simulink model "MODELO_FUZZY"  (R2025b)
settings: Solver=VariableStepAuto  StartTime=0.0  StopTime=30000  RelTol=1e-3
libraries: fuzblock x1
settings Model: PacingRate=1000  Creator=Usuario  LastModifiedBy=Usuario

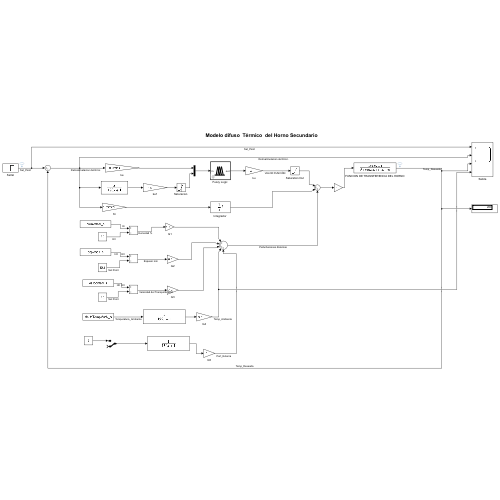
[thumbnail: Simulink's stored preview of the top-level diagram]
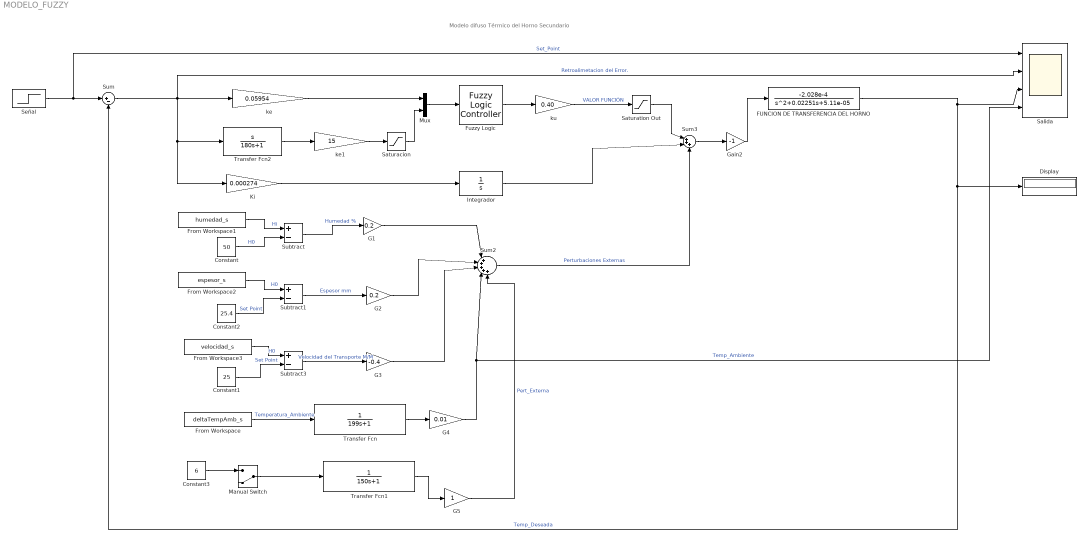
== system MODELO_FUZZY ==
  note: Modelo difuso Térmico del Horno Secundario
  Constant : Constant  Value=50
  Constant1 : Constant  Value=25
  Constant2 : Constant  Value=25.4
  Constant3 : Constant  Value=6
  Display : Display
      settings: Decimation=3
  FUNCION DE TRANSFERENCIA DEL HORNO : TransferFcn  Numerator=[-2.028e-4]  Denominator=[1 0.02251 5.11e-05]
  From Workspace : FromWorkspace  VariableName=deltaTempAmb_s  OutputAfterFinalValue=Holding final value
  From Workspace1 : FromWorkspace  VariableName=humedad_s  OutputAfterFinalValue=Holding final value
  From Workspace2 : FromWorkspace  VariableName=espesor_s  OutputAfterFinalValue=Holding final value
  From Workspace3 : FromWorkspace  VariableName=velocidad_s  OutputAfterFinalValue=Holding final value
  "Fuzzy Logic " : fuzblock/Fuzzy Logic  Controller  FIS='FIS_FB_v5'  OutputSampleNumber=101  DataType=double  UseLookupTable=off  NumBreakpoints=10  FuzzifiedInputs=off  RuleFiringStrengths=off  RuleOutputs=off  AggregatedOutputs=off  SimulateUsing=Interpreted execution  OutOfRangeInputValueMessage=warning  NoRuleFiredMessage=warning  EmptyOutputFuzzySetMessage=warning
  G1 : Gain  Gain=0.2
  G2 : Gain  Gain=0.2
  G3 : Gain  Gain=-0.4
  G4 : Gain  Gain=0.01
  G5 : Gain
  Gain2 : Gain  Gain=-1
  "Integrador " : Integrator  LimitOutput=on  UpperSaturationLimit=1500  LowerSaturationLimit=-1500
  Ki : Gain  Gain=0.000274
  Manual Switch : ManualSwitch  CurrentSetting=0
  Mux : Mux  Inputs=2
  Salida : Scope  NumInputPorts=4
      settings: ActiveDisplayYMinimum=-27.155181326049586  ActiveDisplayYMaximum=227.15518132604959  DataLoggingVariableName=ScopeData2
  "Saturacion " : Saturate  UpperLimit=180  LowerLimit=-180
  Saturation Out : Saturate  UpperLimit=100  LowerLimit=0
  Señal : Step  Time=0  After=200  SampleTime=0
  Subtract : Sum  Inputs=+-
  Subtract1 : Sum  Inputs=+-
  Subtract3 : Sum  Inputs=+-
  Sum : Sum  Inputs=|+-
  Sum2 : Sum  Inputs=|+++++
  Sum3 : Sum  Inputs=|+++
  Transfer Fcn : TransferFcn  Denominator=[199 1]
  Transfer Fcn1 : TransferFcn  Denominator=[150 1]
  Transfer Fcn2 : TransferFcn  Numerator=[1 0]  Denominator=[180 1]
  ke : Gain  Gain=0.05954
  ke1 : Gain  Gain=15
  ku : Gain  Gain=0.40
  wires:
  Señal/1 -> Salida/1, Sum/1  "Set_Point"
  From Workspace1/1 -> Subtract/1  "Hi"
  Transfer Fcn1/1 -> G5/1
  Sum/1 -> ke/1, Salida/2, Ki/1, Transfer Fcn2/1  "Retroalimetacion del Error."
  Constant2/1 -> Subtract1/2  "Set Point"
  Manual Switch/1 -> Transfer Fcn1/1
  Constant/1 -> Subtract/2  "H0"
  Constant1/1 -> Subtract3/2  "Set Point"
  Transfer Fcn/1 -> G4/1
  Subtract1/1 -> G2/1  "Espesor mm"
  From Workspace/1 -> Transfer Fcn/1  "Temperatura_Ambiente"
  Constant3/1 -> Manual Switch/1
  Subtract3/1 -> G3/1  "Velocidad del Transporte M/M"
  From Workspace2/1 -> Subtract1/1  "H0"
  Subtract/1 -> G1/1  "Humedad %"
  ku/1 -> Saturation Out/1  "VALOR FUNCIÓN"
  From Workspace3/1 -> Subtract3/1  "H0"
  "Fuzzy Logic "/1 -> ku/1
  "Saturacion "/1 -> Mux/2
  ke/1 -> Mux/1
  Mux/1 -> "Fuzzy Logic "/1
  Gain2/1 -> FUNCION DE TRANSFERENCIA DEL HORNO/1
  FUNCION DE TRANSFERENCIA DEL HORNO/1 -> Display/1, Sum/2, Salida/3  "Temp_Deseada"
  Saturation Out/1 -> Sum3/1
  Sum3/1 -> Gain2/1
  Sum2/1 -> Sum3/3  "Perturbaciones Externas"
  G1/1 -> Sum2/1
  G2/1 -> Sum2/2
  G3/1 -> Sum2/3
  G4/1 -> Salida/4, Sum2/4  "Temp_Ambiente"
  G5/1 -> Sum2/5  "Pert_Externa"
  Transfer Fcn2/1 -> ke1/1
  ke1/1 -> "Saturacion "/1
  Ki/1 -> "Integrador "/1
  "Integrador "/1 -> Sum3/2
